simulink model "BVH2_App_Layer"  (Simulink 5.1)
settings: Solver=ode45  StartTime=0.0  StopTime=10.0  RelTol=1e-3
PreLoadFcn:
  | if exist('tl_preloadfcn','file'), tl_preloadfcn(gcs,95); end
PostLoadFcn:
  | if exist('tl_postloadfcn','file'), tl_postloadfcn(gcs,95); end
InitFcn:
  | if exist('tlds_start','file'), tlds_start(gcs); end
undefined symbols (not defined in the file): built, constant, Constant, DiscreteIntegrator, Gain, in, Logic, Product, Saturate, Sum, Switch
libraries: tllib x71, simulink x1
(part 3 of 4)

== system BVH2_App_Layer/BVH2_Appl_Layer/Subsystem/SFLogMain ==
  Stateflow Logger : tllib/Extras/Stateflow Logger  data=struct('date',730486)  sflogparam=struct('charts',[16 130 159 276 181 225 101 78 49],'sfblocks',{{'BVH2_App_Layer/BVH2_Appl_Layer/Subsystem/BVH2_Appl_Layer/Current_Analysis_High','BVH2_App_Layer/BVH2_Appl_Layer/Subsystem/BVH2_Appl_Layer/Current_Analysis_low','BVH2_App_Layer/BVH2_Appl_Layer/Subsystem/BVH2_Appl_Layer/Dry_Running','BVH2_App_Layer/BVH2_Appl_Layer/Subsystem/BVH2_Appl_Layer/Dry_RunningAlarm','BVH2_App_Layer/BVH2_Appl_Layer/Subsystem/BVH2_Appl_Layer/Motor_Stalled','BVH2_App_Layer/BVH2_Appl_Layer/Subsystem/BVH2_Appl_Layer/PWM_Detection','BVH2_App_Layer/BVH2_Appl_Layer/Subsystem/BVH2_Appl_Layer/Pic_etat_monitor','BVH2_App_Layer/BVH2_Appl_Layer/Subsystem/BVH2_Appl_Layer/Temperature_Alarm','BVH2_App_Layer/BVH2_Appl_Layer/Subsystem/BVH2_Appl_Layer/UbatHandling'}},'machines',15,'globallogopt',1,'modelname','BVH2_App_Layer','debugmodeactive',1)  flp_block=tldummylib/Stateflow Logger

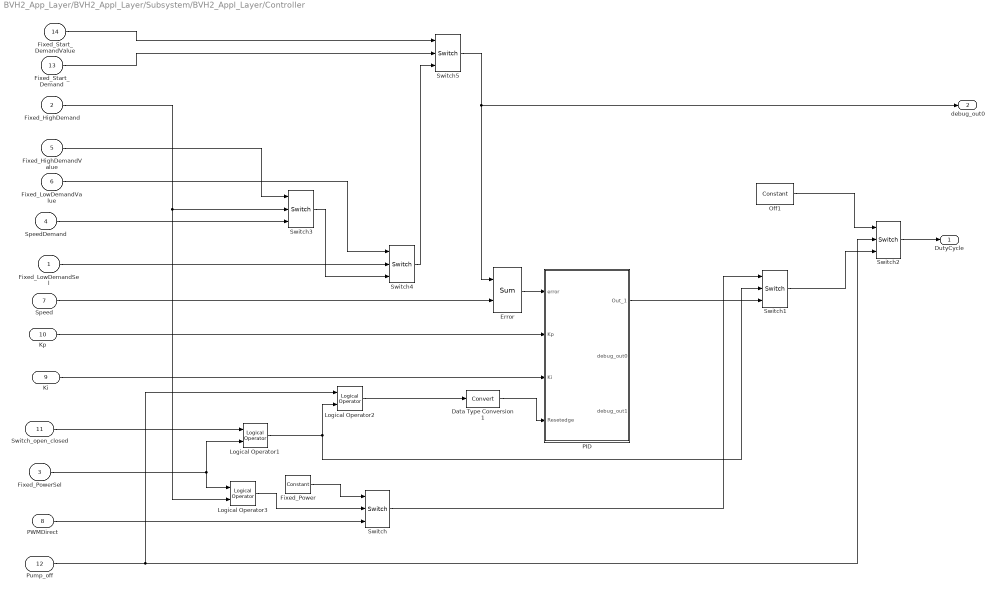
== system BVH2_App_Layer/BVH2_Appl_Layer/Subsystem/BVH2_Appl_Layer/Controller ==
  Fixed_LowDemandSel : Inport  PortDimensions=1  SampleTime=0.01
      settings: CopyFcn=tl_check_ports(gcbh);  NameChangeFcn=tl_check_ports(gcbh);
  Fixed_HighDemand : Inport  Port=2  PortDimensions=1  SampleTime=0.01
      settings: CopyFcn=tl_check_ports(gcbh);  NameChangeFcn=tl_check_ports(gcbh);
  Fixed_PowerSel : Inport  Port=3  PortDimensions=1  SampleTime=0.01
      settings: CopyFcn=tl_check_ports(gcbh);  NameChangeFcn=tl_check_ports(gcbh);
  SpeedDemand : Inport  Port=4  PortDimensions=1  SampleTime=0.01
      settings: CopyFcn=tl_check_ports(gcbh);  NameChangeFcn=tl_check_ports(gcbh);
  Fixed_HighDemandValue : Inport  Port=5  PortDimensions=1  SampleTime=0.01
      settings: CopyFcn=tl_check_ports(gcbh);  NameChangeFcn=tl_check_ports(gcbh);
  Fixed_LowDemandValue : Inport  Port=6  PortDimensions=1  SampleTime=0.01
      settings: CopyFcn=tl_check_ports(gcbh);  NameChangeFcn=tl_check_ports(gcbh);
  Speed : Inport  Port=7  PortDimensions=1  SampleTime=0.01
      settings: CopyFcn=tl_check_ports(gcbh);  NameChangeFcn=tl_check_ports(gcbh);
  PWMDirect : Inport  Port=8  PortDimensions=1  SampleTime=0.01
      settings: CopyFcn=tl_check_ports(gcbh);  NameChangeFcn=tl_check_ports(gcbh);
  Ki : Inport  Port=9  PortDimensions=1  SampleTime=0.01
      settings: CopyFcn=tl_check_ports(gcbh);  NameChangeFcn=tl_check_ports(gcbh);
  Kp : Inport  Port=10  PortDimensions=1  SampleTime=0.01
      settings: CopyFcn=tl_check_ports(gcbh);  NameChangeFcn=tl_check_ports(gcbh);
  Switch_open_closed : Inport  Port=11  PortDimensions=1  SampleTime=0.01
      settings: CopyFcn=tl_check_ports(gcbh);  NameChangeFcn=tl_check_ports(gcbh);
  Pump_off : Inport  Port=12  PortDimensions=1  SampleTime=0.01
      settings: CopyFcn=tl_check_ports(gcbh);  NameChangeFcn=tl_check_ports(gcbh);
  Fixed_Start_Demand : Inport  Port=13  PortDimensions=1  SampleTime=0.01
      settings: CopyFcn=tl_check_ports(gcbh);  NameChangeFcn=tl_check_ports(gcbh);
  Fixed_Start_DemandValue : Inport  Port=14  PortDimensions=1  SampleTime=0.01
      settings: CopyFcn=tl_check_ports(gcbh);  NameChangeFcn=tl_check_ports(gcbh);
  Data Type Conversion1 : DataTypeConversion  SaturateOnIntegerOverflow=on
  Error : tllib/Sum  data=struct('comment',struct('text','','placement',1),'logdata',struct('maxnumvals',inf,'plotchannels',1,'loggingmode',1,'channels',1),'output',struct('width',1,'name','$S_$B','unit','','type','Int16','offset',0,'max',NaN,'min',NaN,'freeze',1,'lsb',1,'arb',0,'class','default','address','','description','','autoscalingmode',1,'lowerheadroom',1,'upperheadroom',1,'headroomunit','bit','checkmin',0,'checkmax',0,'show',0,'variable','','scaling','','keepdatatype',1,'castoutput',0),'inputs','-+','date',735187.627440498,'scalingvalid',0)  lower_limit=1  upper_limit=-1  flp_block=built-in/Sum  help=|
      | Sum block of dSPACE TargetLink.
      | 
      | Output signal is equal to the sum of the input signals.
      | The list of signs is specified according to conventions for Simulink Sum blocks.
  Fixed_Power : tllib/Constant  Value=constant  ShowAdditionalParam=off  OutDataType=sfix(16)  ConRadixGroup=Use specified scaling  OutScaling=2^0  data=struct('comment',struct('text','','placement',1),'output',struct('width',1,'name','$S_$B','unit','','type','UInt16','offset',0,'max',NaN,'min',NaN,'freeze',1,'lsb',1,'arb',0,'class','CONST','address','','description','','value','202','tolerance',1,'show',0,'variable','','scaling','','keepdatatype',1),'date',734643.408264907,'scalingvalid',0)  constant=202  flp_block=built-in/Constant  help=|
      | Constant block of dSPACE TargetLink.
      | 
      | Output signal keeps the given constant value.
  Logical Operator1 : tllib/Logical Operator  data=struct('inputs','2','comment',struct('text','','placement',1),'logdata',struct('maxnumvals',inf,'plotchannels',[],'loggingmode',3,'channels',1),'operator','OR','output',struct('variable','','description','','name','$S_$B','address','','class','default','type','Bool','unit',''),'scalingvalid',0,'date',732283.44913765)  flp_block=built-in/Logic
  Logical Operator2 : tllib/Logical Operator  data=struct('inputs','2','comment',struct('text','','placement',1),'logdata',struct('maxnumvals',inf,'plotchannels',[],'loggingmode',3,'channels',1),'operator','OR','output',struct('variable','','description','','name','$S_$B','address','','class','default','type','Bool','unit',''),'scalingvalid',0,'date',732283.44913765)  flp_block=built-in/Logic
  Logical Operator3 : tllib/Logical Operator  data=struct('inputs','2','comment',struct('text','','placement',1),'logdata',struct('maxnumvals',inf,'plotchannels',[],'loggingmode',3,'channels',1),'operator','OR','output',struct('variable','','description','','name','$S_$B','address','','class','default','type','Bool','unit',''),'scalingvalid',0,'date',732283.44913765)  flp_block=built-in/Logic
  Off1 : tllib/Constant  Value=constant  ShowAdditionalParam=off  OutDataType=sfix(16)  ConRadixGroup=Use specified scaling  OutScaling=2^0  data=struct('comment',struct('text','','placement',1),'output',struct('width',1,'name','$S_$B','unit','','type','Int16','offset',0,'max',NaN,'min',NaN,'freeze',1,'lsb',1,'arb',0,'class','default','address','','description','','value','0','tolerance',1,'show',0,'variable','','scaling','','keepdatatype',1),'date',732121.729407349,'scalingvalid',0)  constant=0  flp_block=built-in/Constant  help=|
      | Constant block of dSPACE TargetLink.
      | 
      | Output signal keeps the given constant value.
  PID : Subsystem
  Switch{,3..5} (4 alike) : tllib/Switch  data=struct('comment',struct('text','','placement',1),'logdata',struct('maxnumvals',inf,'plotchannels',[],'loggingmode',3,'channels',1),'output',struct('variable','','description','','name','$S_$B','width',1,'address','','max',NaN,'min',NaN,'class','default','type','UInt16','scaling','','lsb',1,'offset',0,'arb',0,'freeze',1,'unit','','autoscalingmode',1,'lowerheadroom',1,'upperheadroom',1,'headroomunit','bit','keepdatatype',1,'checkmin',0,'checkmax',0,'castoutput',0,'show',0),'threshold',struct('variable','','description','','name','$S_$B_threshold','width',1,'address','','max',NaN,'min',NaN,'class','default','type','Int16','scaling','','lsb',1,'offset',0,'arb',0,'freeze',1,'unit','','keepdatatype',1,'value','0','scalar',0,'criteria',2),'scalingvalid',0,'date',732283.606852975)  threshold=0  flp_block=built-in/Switch
  Switch1 : tllib/Switch  data=struct('comment',struct('text','','placement',1),'logdata',struct('maxnumvals',inf,'plotchannels',[],'loggingmode',3,'channels',1),'output',struct('variable','','description','','name','$S_$B','width',1,'address','','max',NaN,'min',NaN,'class','default','type','UInt16','scaling','','lsb',1,'offset',0,'arb',0,'freeze',1,'unit','','autoscalingmode',1,'lowerheadroom',1,'upperheadroom',1,'headroomunit','bit','keepdatatype',1,'checkmin',0,'checkmax',0,'castoutput',0,'show',0),'threshold',struct('variable','','description','','name','$S_$B_threshold','width',1,'address','','max',NaN,'min',NaN,'class','default','type','Int16','scaling','','lsb',1,'offset',0,'arb',0,'freeze',1,'unit','','keepdatatype',1,'value','0','scalar',0,'criteria',2),'scalingvalid',0,'date',732283.593361933)  threshold=0  flp_block=built-in/Switch
  Switch2 : tllib/Switch  data=struct('comment',struct('text','','placement',1),'logdata',struct('maxnumvals',inf,'plotchannels',[],'loggingmode',3,'channels',1),'output',struct('variable','','description','','name','$S_$B','width',1,'address','','max',NaN,'min',NaN,'class','default','type','UInt16','scaling','','lsb',1,'offset',0,'arb',0,'freeze',1,'unit','','autoscalingmode',1,'lowerheadroom',1,'upperheadroom',1,'headroomunit','bit','keepdatatype',1,'checkmin',0,'checkmax',0,'castoutput',0,'show',0),'threshold',struct('variable','','description','','name','$S_$B_threshold','width',1,'address','','max',NaN,'min',NaN,'class','default','type','Int16','scaling','','lsb',1,'offset',0,'arb',0,'freeze',1,'unit','','keepdatatype',1,'value','0','scalar',0,'criteria',2),'scalingvalid',0,'date',732289.667383565)  threshold=0  flp_block=built-in/Switch
  DutyCycle : Outport
  debug_out0 : Outport  Port=2
  wires:
  Switch/1 -> Switch1/1
  Error/1 -> PID/1(error)
  Off1/1 -> Switch2/1
  PWMDirect/1 -> Switch/3
  Fixed_PowerSel/1 -> Logical Operator1/2, Logical Operator3/1
  Logical Operator1/1 -> Switch1/2, Logical Operator2/2
  Switch_open_closed/1 -> Logical Operator1/1
  Fixed_Power/1 -> Switch/1
  Pump_off/1 -> Switch2/2, Logical Operator2/1
  Switch1/1 -> Switch2/3
  Data Type Conversion1/1 -> PID/4(Resetedge)
  Logical Operator2/1 -> Data Type Conversion1/1
  Ki/1 -> PID/3(Ki)
  Kp/1 -> PID/2(Kp)
  PID/1(Out_1) -> Switch1/3
  Switch2/1 -> DutyCycle/1
  Speed/1 -> Error/2
  Fixed_HighDemand/1 -> Switch3/2, Logical Operator3/2
  Fixed_HighDemandValue/1 -> Switch3/1
  Logical Operator3/1 -> Switch/2
  Switch3/1 -> Switch4/3
  Fixed_LowDemandSel/1 -> Switch4/2
  Fixed_LowDemandValue/1 -> Switch4/1
  Fixed_Start_DemandValue/1 -> Switch5/1
  Fixed_Start_Demand/1 -> Switch5/2
  SpeedDemand/1 -> Switch3/3
  Switch4/1 -> Switch5/3
  Switch5/1 -> debug_out0/1, Error/1

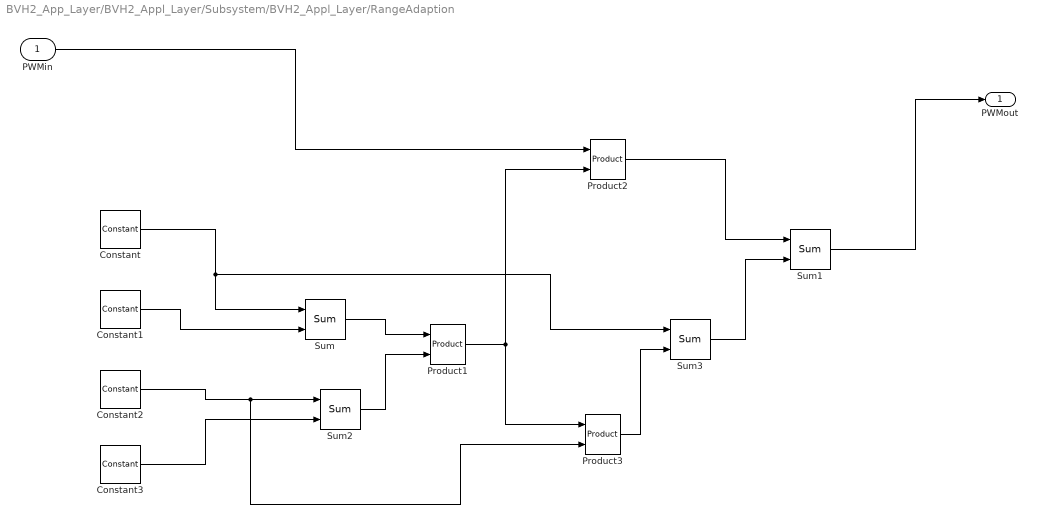
== system BVH2_App_Layer/BVH2_Appl_Layer/Subsystem/BVH2_Appl_Layer/RangeAdaption ==
  PWMin : Inport  PortDimensions=1  SampleTime=0.01
      settings: CopyFcn=tl_check_ports(gcbh);  NameChangeFcn=tl_check_ports(gcbh);
  Constant : tllib/Constant  Value=constant  ShowAdditionalParam=off  OutDataType=sfix(16)  ConRadixGroup=Use specified scaling  OutScaling=2^0  data=struct('comment',struct('text','','placement',1),'output',struct('variable','','description','','name','$S_$B','width',1,'address','','max',NaN,'min',NaN,'class','default','type','Int16','scaling','','lsb',1,'offset',0,'arb',0,'freeze',1,'unit','','keepdatatype',1,'value','200','tolerance',1,'show',0),'dt','inf','scalingvalid',0,'date',734591.489153391)  constant=200  flp_block=built-in/Constant
  Constant1 : tllib/Constant  Value=constant  ShowAdditionalParam=off  OutDataType=sfix(16)  ConRadixGroup=Use specified scaling  OutScaling=2^0  data=struct('comment',struct('text','','placement',1),'output',struct('variable','','description','','name','$S_$B','width',1,'address','','max',NaN,'min',NaN,'class','default','type','Int16','scaling','','lsb',1,'offset',0,'arb',0,'freeze',1,'unit','','keepdatatype',1,'value','60','tolerance',1,'show',0),'dt','inf','scalingvalid',0,'date',734591.489234537)  constant=60  flp_block=built-in/Constant
  Constant2 : tllib/Constant  Value=constant  ShowAdditionalParam=off  OutDataType=sfix(16)  ConRadixGroup=Use specified scaling  OutScaling=2^0  data=struct('comment',struct('text','','placement',1),'output',struct('variable','','description','','name','$S_$B','width',1,'address','','max',NaN,'min',NaN,'class','default','type','Int16','scaling','','lsb',1,'offset',0,'arb',0,'freeze',1,'unit','','keepdatatype',1,'value','190','tolerance',1,'show',0),'dt','inf','scalingvalid',0,'date',734591.488197627)  constant=190  flp_block=built-in/Constant
  Constant3 : tllib/Constant  Value=constant  ShowAdditionalParam=off  OutDataType=sfix(16)  ConRadixGroup=Use specified scaling  OutScaling=2^0  data=struct('comment',struct('text','','placement',1),'output',struct('variable','','description','','name','$S_$B','width',1,'address','','max',NaN,'min',NaN,'class','default','type','Int16','scaling','','lsb',1,'offset',0,'arb',0,'freeze',1,'unit','','keepdatatype',1,'value','30','tolerance',1,'show',0),'dt','inf','scalingvalid',0,'date',734591.48794713)  constant=30  flp_block=built-in/Constant
  Product1 : tllib/Product  data=struct('comment',struct('text','','placement',1),'logdata',struct('maxnumvals',inf,'plotchannels',[],'loggingmode',3,'channels',1),'output',struct('width',1,'name','$S_$B','unit','','type','UInt16','offset',0,'max',NaN,'min',NaN,'freeze',1,'lsb',2^-8,'arb',0,'class','default','address','','description','','autoscalingmode',1,'lowerheadroom',0,'upperheadroom',1,'headroomunit','bit','checkmin',0,'checkmax',0,'show',0,'variable','','scaling','','keepdatatype',1,'castoutput',0),'inputs','*/','exceptionhandling',1,'date',734591.551719815,'scalingvalid',0)  lower_limit=1  upper_limit=-1  flp_block=built-in/Product  help=|
      | Product block of dSPACE TargetLink.
      | 
      | Output signal is equal to the product of the input signals. The input ports are specified according to conventions for Simulink Product blocks.
  Product2 : tllib/Product  data=struct('comment',struct('text','','placement',1),'logdata',struct('maxnumvals',inf,'plotchannels',[],'loggingmode',3,'channels',1),'output',struct('width',1,'name','$S_$B','unit','','type','UInt16','offset',0,'max',NaN,'min',NaN,'freeze',1,'lsb',1,'arb',0,'class','default','address','','description','','autoscalingmode',1,'lowerheadroom',0,'upperheadroom',1,'headroomunit','bit','checkmin',0,'checkmax',0,'show',0,'variable','','scaling','','keepdatatype',1,'castoutput',0),'inputs','**','exceptionhandling',1,'date',732813.755751852,'scalingvalid',0)  lower_limit=1  upper_limit=-1  flp_block=built-in/Product  help=|
      | Product block of dSPACE TargetLink.
      | 
      | Output signal is equal to the product of the input signals. The input ports are specified according to conventions for Simulink Product blocks.
  Product3 : tllib/Product  data=struct('comment',struct('text','','placement',1),'logdata',struct('maxnumvals',inf,'plotchannels',[],'loggingmode',3,'channels',1),'output',struct('width',1,'name','$S_$B','unit','','type','UInt16','offset',0,'max',NaN,'min',NaN,'freeze',1,'lsb',1,'arb',0,'class','default','address','','description','','autoscalingmode',1,'lowerheadroom',0,'upperheadroom',1,'headroomunit','bit','checkmin',0,'checkmax',0,'show',0,'variable','','scaling','','keepdatatype',1,'castoutput',0),'inputs','**','exceptionhandling',1,'date',732813.755751852,'scalingvalid',0)  lower_limit=1  upper_limit=-1  flp_block=built-in/Product  help=|
      | Product block of dSPACE TargetLink.
      | 
      | Output signal is equal to the product of the input signals. The input ports are specified according to conventions for Simulink Product blocks.
  Sum : tllib/Sum  data=struct('comment',struct('text','','placement',1),'logdata',struct('maxnumvals',inf,'plotchannels',[],'loggingmode',3,'channels',1),'output',struct('variable','','description','','name','$S_$B','width',1,'address','','max',NaN,'min',NaN,'class','default','type','Int16','scaling','','lsb',1,'offset',0,'arb',0,'freeze',1,'unit','','autoscalingmode',1,'lowerheadroom',1,'upperheadroom',1,'headroomunit','bit','keepdatatype',1,'checkmin',0,'checkmax',0,'castoutput',0,'show',0),'inputs','+-','scalingvalid',0,'date',733019.586384155)  flp_block=built-in/Sum
  Sum1 : tllib/Sum  data=struct('comment',struct('text','','placement',1),'logdata',struct('maxnumvals',inf,'plotchannels',[],'loggingmode',3,'channels',1),'output',struct('variable','','description','','name','$S_$B','width',1,'address','','max',NaN,'min',NaN,'class','default','type','Int16','scaling','','lsb',1,'offset',0,'arb',0,'freeze',1,'unit','','autoscalingmode',1,'lowerheadroom',1,'upperheadroom',1,'headroomunit','bit','keepdatatype',1,'checkmin',0,'checkmax',0,'castoutput',0,'show',0),'inputs','++','scalingvalid',0,'date',734591.551219225)  flp_block=built-in/Sum
  Sum2 : tllib/Sum  data=struct('comment',struct('text','','placement',1),'logdata',struct('maxnumvals',inf,'plotchannels',[],'loggingmode',3,'channels',1),'output',struct('variable','','description','','name','$S_$B','width',1,'address','','max',NaN,'min',NaN,'class','default','type','Int16','scaling','','lsb',1,'offset',0,'arb',0,'freeze',1,'unit','','autoscalingmode',1,'lowerheadroom',1,'upperheadroom',1,'headroomunit','bit','keepdatatype',1,'checkmin',0,'checkmax',0,'castoutput',0,'show',0),'inputs','+-','scalingvalid',0,'date',733019.586384155)  flp_block=built-in/Sum
  Sum3 : tllib/Sum  data=struct('comment',struct('text','','placement',1),'logdata',struct('maxnumvals',inf,'plotchannels',[],'loggingmode',3,'channels',1),'output',struct('variable','','description','','name','$S_$B','width',1,'address','','max',NaN,'min',NaN,'class','default','type','Int16','scaling','','lsb',1,'offset',0,'arb',0,'freeze',1,'unit','','autoscalingmode',1,'lowerheadroom',1,'upperheadroom',1,'headroomunit','bit','keepdatatype',1,'checkmin',0,'checkmax',0,'castoutput',0,'show',0),'inputs','+-','scalingvalid',0,'date',733019.586384155)  flp_block=built-in/Sum
  PWMout : Outport
  wires:
  PWMin/1 -> Product2/1
  Product2/1 -> Sum1/1
  Constant/1 -> Sum/1, Sum3/1
  Constant1/1 -> Sum/2
  Sum/1 -> Product1/1
  Constant2/1 -> Sum2/1, Product3/2
  Constant3/1 -> Sum2/2
  Sum2/1 -> Product1/2
  Product1/1 -> Product2/2, Product3/1
  Product3/1 -> Sum3/2
  Sum3/1 -> Sum1/2
  Sum1/1 -> PWMout/1

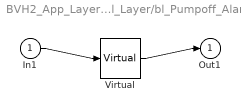
== system BVH2_App_Layer/BVH2_Appl_Layer/Subsystem/BVH2_Appl_Layer/bl_Pumpoff_Alarm ==
  In1 : Inport
  Virtual : tllib/Virtual  SimViewingDevice=off  DataTypeOverride=UseLocalSettings  MinMaxOverflowLogging=UseLocalSettings
      settings: Permissions=ReadWrite  RTWFcnNameOpts=Auto  RTWFileNameOpts=Auto
  Out1 : Outport
  wires:
  In1/1 -> Virtual/1
  Virtual/1 -> Out1/1

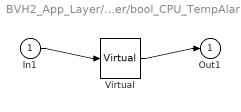
== system BVH2_App_Layer/BVH2_Appl_Layer/Subsystem/BVH2_Appl_Layer/bool_CPU_TempAlarm ==
  In1 : Inport
  Virtual : tllib/Virtual  SimViewingDevice=off  DataTypeOverride=UseLocalSettings  MinMaxOverflowLogging=UseLocalSettings
      settings: Permissions=ReadWrite  RTWFcnNameOpts=Auto  RTWFileNameOpts=Auto
  Out1 : Outport
  wires:
  In1/1 -> Virtual/1
  Virtual/1 -> Out1/1

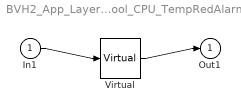
== system BVH2_App_Layer/BVH2_Appl_Layer/Subsystem/BVH2_Appl_Layer/bool_CPU_TempRedAlarm ==
  In1 : Inport
  Virtual : tllib/Virtual  SimViewingDevice=off  DataTypeOverride=UseLocalSettings  MinMaxOverflowLogging=UseLocalSettings
      settings: Permissions=ReadWrite  RTWFcnNameOpts=Auto  RTWFileNameOpts=Auto
  Out1 : Outport
  wires:
  In1/1 -> Virtual/1
  Virtual/1 -> Out1/1

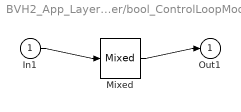
== system BVH2_App_Layer/BVH2_Appl_Layer/Subsystem/BVH2_Appl_Layer/bool_ControlLoopMode ==
  In1 : Inport
  Mixed : tllib/Mixed  SimViewingDevice=off  DataTypeOverride=UseLocalSettings  MinMaxOverflowLogging=UseLocalSettings
      settings: Permissions=ReadWrite  RTWFcnNameOpts=Auto  RTWFileNameOpts=Auto
  Out1 : Outport
  wires:
  In1/1 -> Mixed/1
  Mixed/1 -> Out1/1

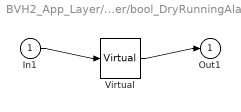
== system BVH2_App_Layer/BVH2_Appl_Layer/Subsystem/BVH2_Appl_Layer/bool_DryRunningAlarm ==
  In1 : Inport
  Virtual : tllib/Virtual  SimViewingDevice=off  DataTypeOverride=UseLocalSettings  MinMaxOverflowLogging=UseLocalSettings
      settings: Permissions=ReadWrite  RTWFcnNameOpts=Auto  RTWFileNameOpts=Auto
  Out1 : Outport
  wires:
  In1/1 -> Virtual/1
  Virtual/1 -> Out1/1

== system BVH2_App_Layer/BVH2_Appl_Layer/Subsystem/BVH2_Appl_Layer/bool_HighCurrentAlarm ==
  In1 : Inport
  Virtual : tllib/Virtual  SimViewingDevice=off  DataTypeOverride=UseLocalSettings  MinMaxOverflowLogging=UseLocalSettings
      settings: Permissions=ReadWrite  RTWFcnNameOpts=Auto  RTWFileNameOpts=Auto
  Out1 : Outport
  wires:
  In1/1 -> Virtual/1
  Virtual/1 -> Out1/1

== system BVH2_App_Layer/BVH2_Appl_Layer/Subsystem/BVH2_Appl_Layer/bool_MotorStalled ==
  In1 : Inport
  Virtual : tllib/Virtual  SimViewingDevice=off  DataTypeOverride=UseLocalSettings  MinMaxOverflowLogging=UseLocalSettings
      settings: Permissions=ReadWrite  RTWFcnNameOpts=Auto  RTWFileNameOpts=Auto
  Out1 : Outport
  wires:
  In1/1 -> Virtual/1
  Virtual/1 -> Out1/1

== system BVH2_App_Layer/BVH2_Appl_Layer/Subsystem/BVH2_Appl_Layer/bool_PIC_Alarm ==
  In1 : Inport
  Virtual : tllib/Virtual  SimViewingDevice=off  DataTypeOverride=UseLocalSettings  MinMaxOverflowLogging=UseLocalSettings
      settings: Permissions=ReadWrite  RTWFcnNameOpts=Auto  RTWFileNameOpts=Auto
  Out1 : Outport
  wires:
  In1/1 -> Virtual/1
  Virtual/1 -> Out1/1

== system BVH2_App_Layer/BVH2_Appl_Layer/Subsystem/BVH2_Appl_Layer/bool_PWMin_Freq_err_Alarm ==
  In1 : Inport
  Virtual : tllib/Virtual  SimViewingDevice=off  DataTypeOverride=UseLocalSettings  MinMaxOverflowLogging=UseLocalSettings
      settings: Permissions=ReadWrite  RTWFcnNameOpts=Auto  RTWFileNameOpts=Auto
  Out1 : Outport
  wires:
  In1/1 -> Virtual/1
  Virtual/1 -> Out1/1

== system BVH2_App_Layer/BVH2_Appl_Layer/Subsystem/BVH2_Appl_Layer/bool_PWMin_err_Alarm ==
  In1 : Inport
  Virtual : tllib/Virtual  SimViewingDevice=off  DataTypeOverride=UseLocalSettings  MinMaxOverflowLogging=UseLocalSettings
      settings: Permissions=ReadWrite  RTWFcnNameOpts=Auto  RTWFileNameOpts=Auto
  Out1 : Outport
  wires:
  In1/1 -> Virtual/1
  Virtual/1 -> Out1/1

== system BVH2_App_Layer/BVH2_Appl_Layer/Subsystem/BVH2_Appl_Layer/bool_StalledMotorStop ==
  In1 : Inport
  Virtual : tllib/Virtual  SimViewingDevice=off  DataTypeOverride=UseLocalSettings  MinMaxOverflowLogging=UseLocalSettings
      settings: Permissions=ReadWrite  RTWFcnNameOpts=Auto  RTWFileNameOpts=Auto
  Out1 : Outport
  wires:
  In1/1 -> Virtual/1
  Virtual/1 -> Out1/1

== system BVH2_App_Layer/BVH2_Appl_Layer/Subsystem/BVH2_Appl_Layer/bool_UbatAlarm ==
  In1 : Inport
  Virtual : tllib/Virtual  SimViewingDevice=off  DataTypeOverride=UseLocalSettings  MinMaxOverflowLogging=UseLocalSettings
      settings: Permissions=ReadWrite  RTWFcnNameOpts=Auto  RTWFileNameOpts=Auto
  Out1 : Outport
  wires:
  In1/1 -> Virtual/1
  Virtual/1 -> Out1/1

== system BVH2_App_Layer/BVH2_Appl_Layer/Subsystem/BVH2_Appl_Layer/bool_mat_currAlarm_bldc ==
  In1 : Inport
  Mixed : tllib/Mixed  SimViewingDevice=off  DataTypeOverride=UseLocalSettings  MinMaxOverflowLogging=UseLocalSettings
      settings: Permissions=ReadWrite  RTWFcnNameOpts=Auto  RTWFileNameOpts=Auto
  Out1 : Outport
  wires:
  In1/1 -> Mixed/1
  Mixed/1 -> Out1/1

== system BVH2_App_Layer/BVH2_Appl_Layer/Subsystem/BVH2_Appl_Layer/bool_mat_pic_etat ==
  In1 : Inport
  Mixed : tllib/Mixed  SimViewingDevice=off  DataTypeOverride=UseLocalSettings  MinMaxOverflowLogging=UseLocalSettings
      settings: Permissions=ReadWrite  RTWFcnNameOpts=Auto  RTWFileNameOpts=Auto
  Out1 : Outport
  wires:
  In1/1 -> Mixed/1
  Mixed/1 -> Out1/1

== system BVH2_App_Layer/BVH2_Appl_Layer/Subsystem/BVH2_Appl_Layer/bool_start_demand_mat ==
  In1 : Inport
  Mixed : tllib/Mixed  SimViewingDevice=off  DataTypeOverride=UseLocalSettings  MinMaxOverflowLogging=UseLocalSettings
      settings: Permissions=ReadWrite  RTWFcnNameOpts=Auto  RTWFileNameOpts=Auto
  Out1 : Outport
  wires:
  In1/1 -> Mixed/1
  Mixed/1 -> Out1/1

== system BVH2_App_Layer/BVH2_Appl_Layer/Subsystem/BVH2_Appl_Layer/ui16_Current_Thresh ==
  In1 : Inport
  Mixed : tllib/Mixed  SimViewingDevice=off  DataTypeOverride=UseLocalSettings  MinMaxOverflowLogging=UseLocalSettings
      settings: Permissions=ReadWrite  RTWFcnNameOpts=Auto  RTWFileNameOpts=Auto
  Out1 : Outport
  wires:
  In1/1 -> Mixed/1
  Mixed/1 -> Out1/1

== system BVH2_App_Layer/BVH2_Appl_Layer/Subsystem/BVH2_Appl_Layer/ui16_PWM_Freq_mat ==
  In1 : Inport
  Mixed : tllib/Mixed  SimViewingDevice=off  DataTypeOverride=UseLocalSettings  MinMaxOverflowLogging=UseLocalSettings
      settings: Permissions=ReadWrite  RTWFcnNameOpts=Auto  RTWFileNameOpts=Auto
  Out1 : Outport
  wires:
  In1/1 -> Mixed/1
  Mixed/1 -> Out1/1

== system BVH2_App_Layer/BVH2_Appl_Layer/Subsystem/BVH2_Appl_Layer/ui16_Speed_demand_mat ==
  In1 : Inport
  Mixed : tllib/Mixed  SimViewingDevice=off  DataTypeOverride=UseLocalSettings  MinMaxOverflowLogging=UseLocalSettings
      settings: Permissions=ReadWrite  RTWFcnNameOpts=Auto  RTWFileNameOpts=Auto
  Out1 : Outport
  wires:
  In1/1 -> Mixed/1
  Mixed/1 -> Out1/1

== system BVH2_App_Layer/BVH2_Appl_Layer/Subsystem/BVH2_Appl_Layer/ui16_Speed_demand_mat_Max ==
  In1 : Inport
  Mixed : tllib/Mixed  SimViewingDevice=off  DataTypeOverride=UseLocalSettings  MinMaxOverflowLogging=UseLocalSettings
      settings: Permissions=ReadWrite  RTWFcnNameOpts=Auto  RTWFileNameOpts=Auto
  Out1 : Outport
  wires:
  In1/1 -> Mixed/1
  Mixed/1 -> Out1/1

== system BVH2_App_Layer/BVH2_Appl_Layer/Subsystem/BVH2_Appl_Layer/ui16_Speed_demand_mat_min ==
  In1 : Inport
  Mixed : tllib/Mixed  SimViewingDevice=off  DataTypeOverride=UseLocalSettings  MinMaxOverflowLogging=UseLocalSettings
      settings: Permissions=ReadWrite  RTWFcnNameOpts=Auto  RTWFileNameOpts=Auto
  Out1 : Outport
  wires:
  In1/1 -> Mixed/1
  Mixed/1 -> Out1/1

== system BVH2_App_Layer/BVH2_Appl_Layer/Subsystem/BVH2_Appl_Layer/ui16_Speed_mat ==
  In1 : Inport
  Mixed : tllib/Mixed  SimViewingDevice=off  DataTypeOverride=UseLocalSettings  MinMaxOverflowLogging=UseLocalSettings
      settings: Permissions=ReadWrite  RTWFcnNameOpts=Auto  RTWFileNameOpts=Auto
  Out1 : Outport
  wires:
  In1/1 -> Mixed/1
  Mixed/1 -> Out1/1

== system BVH2_App_Layer/BVH2_Appl_Layer/Subsystem/BVH2_Appl_Layer/ui16_dryRun_Thresh ==
  In1 : Inport
  Mixed : tllib/Mixed  SimViewingDevice=off  DataTypeOverride=UseLocalSettings  MinMaxOverflowLogging=UseLocalSettings
      settings: Permissions=ReadWrite  RTWFcnNameOpts=Auto  RTWFileNameOpts=Auto
  Out1 : Outport
  wires:
  In1/1 -> Mixed/1
  Mixed/1 -> Out1/1

== system BVH2_App_Layer/BVH2_Appl_Layer/Subsystem/BVH2_Appl_Layer/ui16_mat_Current ==
  In1 : Inport
  Mixed : tllib/Mixed  SimViewingDevice=off  DataTypeOverride=UseLocalSettings  MinMaxOverflowLogging=UseLocalSettings
      settings: Permissions=ReadWrite  RTWFcnNameOpts=Auto  RTWFileNameOpts=Auto
  Out1 : Outport
  wires:
  In1/1 -> Mixed/1
  Mixed/1 -> Out1/1

== system BVH2_App_Layer/BVH2_Appl_Layer/Subsystem/BVH2_Appl_Layer/ui16_mat_inpTemp ==
  In1 : Inport
  Mixed : tllib/Mixed  SimViewingDevice=off  DataTypeOverride=UseLocalSettings  MinMaxOverflowLogging=UseLocalSettings
      settings: Permissions=ReadWrite  RTWFcnNameOpts=Auto  RTWFileNameOpts=Auto
  Out1 : Outport
  wires:
  In1/1 -> Mixed/1
  Mixed/1 -> Out1/1

== system BVH2_App_Layer/BVH2_Appl_Layer/Subsystem/BVH2_Appl_Layer/ui8_BattVolt_mat ==
  In1 : Inport
  Mixed : tllib/Mixed  SimViewingDevice=off  DataTypeOverride=UseLocalSettings  MinMaxOverflowLogging=UseLocalSettings
      settings: Permissions=ReadWrite  RTWFcnNameOpts=Auto  RTWFileNameOpts=Auto
  Out1 : Outport
  wires:
  In1/1 -> Mixed/1
  Mixed/1 -> Out1/1

== system BVH2_App_Layer/BVH2_Appl_Layer/Subsystem/BVH2_Appl_Layer/ui8_Ki_mat ==
  In1 : Inport
  Mixed : tllib/Mixed  SimViewingDevice=off  DataTypeOverride=UseLocalSettings  MinMaxOverflowLogging=UseLocalSettings
      settings: Permissions=ReadWrite  RTWFcnNameOpts=Auto  RTWFileNameOpts=Auto
  Out1 : Outport
  wires:
  In1/1 -> Mixed/1
  Mixed/1 -> Out1/1

== system BVH2_App_Layer/BVH2_Appl_Layer/Subsystem/BVH2_Appl_Layer/ui8_Kp_mat ==
  In1 : Inport
  Mixed : tllib/Mixed  SimViewingDevice=off  DataTypeOverride=UseLocalSettings  MinMaxOverflowLogging=UseLocalSettings
      settings: Permissions=ReadWrite  RTWFcnNameOpts=Auto  RTWFileNameOpts=Auto
  Out1 : Outport
  wires:
  In1/1 -> Mixed/1
  Mixed/1 -> Out1/1

== system BVH2_App_Layer/BVH2_Appl_Layer/Subsystem/BVH2_Appl_Layer/ui8_PWM_dc_mat ==
  In1 : Inport
  Mixed : tllib/Mixed  SimViewingDevice=off  DataTypeOverride=UseLocalSettings  MinMaxOverflowLogging=UseLocalSettings
      settings: Permissions=ReadWrite  RTWFcnNameOpts=Auto  RTWFileNameOpts=Auto
  Out1 : Outport
  wires:
  In1/1 -> Mixed/1
  Mixed/1 -> Out1/1

== system BVH2_App_Layer/BVH2_Appl_Layer/Subsystem/BVH2_Appl_Layer/ui8_ResetMatlab ==
  In1 : Inport
  Mixed : tllib/Mixed  SimViewingDevice=off  DataTypeOverride=UseLocalSettings  MinMaxOverflowLogging=UseLocalSettings
      settings: Permissions=ReadWrite  RTWFcnNameOpts=Auto  RTWFileNameOpts=Auto
  Out1 : Outport
  wires:
  In1/1 -> Mixed/1
  Mixed/1 -> Out1/1

== system BVH2_App_Layer/BVH2_Appl_Layer/Subsystem/BVH2_Appl_Layer/ui8_debug_out0 ==
  In1 : Inport
  Virtual : tllib/Virtual  SimViewingDevice=off  DataTypeOverride=UseLocalSettings  MinMaxOverflowLogging=UseLocalSettings
      settings: Permissions=ReadWrite  RTWFcnNameOpts=Auto  RTWFileNameOpts=Auto
  Out1 : Outport
  wires:
  In1/1 -> Virtual/1
  Virtual/1 -> Out1/1

== system BVH2_App_Layer/BVH2_Appl_Layer/Subsystem/BVH2_Appl_Layer/ui8_duty_cycle_mat ==
  In1 : Inport
  Virtual : tllib/Virtual  SimViewingDevice=off  DataTypeOverride=UseLocalSettings  MinMaxOverflowLogging=UseLocalSettings
      settings: Permissions=ReadWrite  RTWFcnNameOpts=Auto  RTWFileNameOpts=Auto
  Out1 : Outport
  wires:
  In1/1 -> Virtual/1
  Virtual/1 -> Out1/1

== system BVH2_App_Layer/BVH2_Appl_Layer/Subsystem/BVH2_Appl_Layer/ui8_fixed_start_speed_mat ==
  In1 : Inport
  Mixed : tllib/Mixed  SimViewingDevice=off  DataTypeOverride=UseLocalSettings  MinMaxOverflowLogging=UseLocalSettings
      settings: Permissions=ReadWrite  RTWFcnNameOpts=Auto  RTWFileNameOpts=Auto
  Out1 : Outport
  wires:
  In1/1 -> Mixed/1
  Mixed/1 -> Out1/1

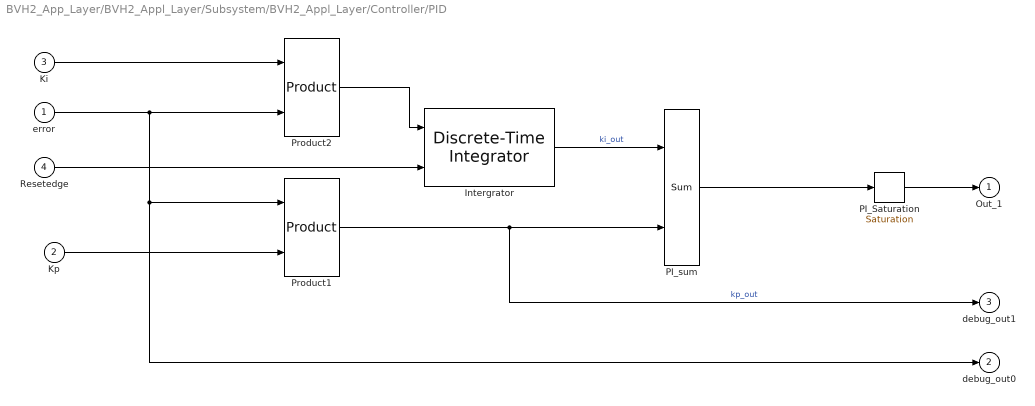
== system BVH2_App_Layer/BVH2_Appl_Layer/Subsystem/BVH2_Appl_Layer/Controller/PID ==
  error : Inport
  Kp : Inport  Port=2
  Ki : Inport  Port=3
  Resetedge : Inport  Port=4
  Intergrator : tllib/Discrete-Time Integrator  data=struct('comment',struct('text','','placement',1),'logdata',struct('maxnumvals',inf,'plotchannels',[],'loggingmode',3,'channels',1),'output',struct('width',1,'name','$S_$B','unit','','type','Int16','offset',0,'max',NaN,'min',NaN,'freeze',1,'lsb',1,'arb',0,'class','default','address','','description','','autoscalingmode',1,'lowerheadroom',1,'upperheadroom',1,'headroomunit','bit','show',0,'variable','','scaling','','keepdatatype',1,'castoutput',1),'state',struct('width',1,'name','X_$S_$B','unit','','type','Int16','offset',0,'max',NaN,'min',NaN,'freeze',1,'lsb',1,'arb',0,'class','default','address','','description','','externalreset',4,'initialconditionsource',1,'showsaturation',0,'initial','100','variable','','scaling',''),'input',struct('name','U_$S_$B','unit','','class','default','address','','description','','variable',''),'lowerlimit',struct('width',1,'name','$S_$B_lower','unit','','type','Int16','offset',0,'max',NaN,'min',NaN,'freeze',1,'lsb',1,'arb',0,'class','default','address','','description','','value','40','variable','','scaling','','keepdatatype',1),'upperlimit',struct('width',1,'name','$S_$B_upper','unit','','type','Int16','offset',0,'max',NaN,'min',NaN,'freeze',1,'lsb',1,'arb',0,'class','default','address','','description','','value','202','variable','','scaling','','keepdatatype',1),'integrationmethod',1,'dt','0.01','date',734772.541916007,'scalingvalid',0)  dt=0.01  lower_limit=40  upper_limit=202  X0=100  flp_block=built-in/DiscreteIntegrator  help=|
      | Discrete Integrator block of dSPACE TargetLink.
      | Forward and backward rectangular and trapezoidal integration are supported.
      | 
      | Note that this block is not vectorized.
  PI_Saturation : tllib/Saturation  data=struct('comment',struct('text','','placement',1),'logdata',struct('maxnumvals',inf,'plotchannels',[],'loggingmode',3,'channels',1),'output',struct('width',1,'name','$S_$B','unit','','type','UInt16','offset',0,'max',NaN,'min',NaN,'freeze',1,'lsb',1,'arb',0,'class','default','address','','description','','autoscalingmode',1,'lowerheadroom',0,'upperheadroom',1,'headroomunit','bit','show',0,'variable','','scaling','','keepdatatype',1,'castoutput',0),'lowerlimit',struct('width',1,'name','$S_$B_lower','unit','','type','Int16','offset',0,'max',NaN,'min',NaN,'freeze',1,'lsb',1,'arb',0,'class','default','address','','description','','value','40','scalar',0,'variable','','scaling','','keepdatatype',1),'upperlimit',struct('width',1,'name','$S_$B_upper','unit','','type','Int16','offset',0,'max',NaN,'min',NaN,'freeze',1,'lsb',1,'arb',0,'class','default','address','','description','','value','202','scalar',0,'variable','','scaling','','keepdatatype',1),'date',734772.541953438,'scalingvalid',0)  lower_limit=40  upper_limit=202  flp_block=built-in/Saturate  help=|
      | Saturation block of dSPACE TargetLink.
      | 
      | The Saturation block saturates its input to the given upper and lower limit.
  PI_sum : tllib/Sum  data=struct('comment',struct('text','','placement',1),'logdata',struct('maxnumvals',inf,'plotchannels',[],'loggingmode',3,'channels',1),'output',struct('width',1,'name','$S_$B','unit','','type','Int16','offset',0,'max',NaN,'min',NaN,'freeze',1,'lsb',1,'arb',0,'class','default','address','','description','','autoscalingmode',1,'lowerheadroom',1,'upperheadroom',1,'headroomunit','bit','checkmin',0,'checkmax',0,'show',0,'variable','','scaling','','keepdatatype',1,'castoutput',0),'inputs','++','date',734643.573882407,'scalingvalid',0)  lower_limit=1  upper_limit=-1  flp_block=built-in/Sum  help=|
      | Sum block of dSPACE TargetLink.
      | 
      | Output signal is equal to the sum of the input signals.
      | The list of signs is specified according to conventions for Simulink Sum blocks.
  Product1 : tllib/Product  data=struct('comment',struct('text','','placement',1),'logdata',struct('maxnumvals',inf,'plotchannels',[],'loggingmode',3,'channels',1),'output',struct('width',1,'name','$S_$B','unit','','type','Int16','offset',0,'max',NaN,'min',NaN,'freeze',1,'lsb',1,'arb',0,'class','default','address','','description','','autoscalingmode',1,'lowerheadroom',1,'upperheadroom',1,'headroomunit','bit','checkmin',0,'checkmax',0,'show',0,'variable','','scaling','','keepdatatype',1,'castoutput',0),'inputs','**','exceptionhandling',1,'date',734643.573922176,'scalingvalid',0)  lower_limit=1  upper_limit=-1  flp_block=built-in/Product  help=|
      | Product block of dSPACE TargetLink.
      | 
      | Output signal is equal to the product of the input signals. The input ports are specified according to conventions for Simulink Product blocks.
  Product2 : tllib/Product  data=struct('comment',struct('text','','placement',1),'logdata',struct('maxnumvals',inf,'plotchannels',[],'loggingmode',3,'channels',1),'output',struct('width',1,'name','$S_$B','unit','','type','Int16','offset',0,'max',NaN,'min',NaN,'freeze',1,'lsb',2^-3,'arb',0,'class','default','address','','description','','autoscalingmode',1,'lowerheadroom',1,'upperheadroom',1,'headroomunit','bit','checkmin',0,'checkmax',0,'show',0,'variable','','scaling','','keepdatatype',1,'castoutput',0),'inputs','**','exceptionhandling',1,'date',734713.639518102,'scalingvalid',0)  lower_limit=1  upper_limit=-1  flp_block=built-in/Product  help=|
      | Product block of dSPACE TargetLink.
      | 
      | Output signal is equal to the product of the input signals. The input ports are specified according to conventions for Simulink Product blocks.
  Out_1 : Outport  InitialOutput=0
  debug_out0 : Outport  Port=2  InitialOutput=0
  debug_out1 : Outport  Port=3  InitialOutput=0
  wires:
  error/1 -> Product2/2, Product1/1, debug_out0/1
  Product2/1 -> Intergrator/1
  Intergrator/1 -> PI_sum/1  "ki_out"
  Kp/1 -> Product1/2
  Ki/1 -> Product2/1
  PI_Saturation/1 -> Out_1/1
  Resetedge/1 -> Intergrator/2
  PI_sum/1 -> PI_Saturation/1
  Product1/1 -> PI_sum/2, debug_out1/1  "kp_out"

== stateflow chart BVH2_Appl_Layer/Subsystem/BVH2_Appl_Layer/Current_Analysis_High ==
  state redState
    entry:
    StateCnt=0;
    oShutoff = 1;
    oCurrentAlarm = 1;
    during:
    StateCnt++;
  state CntOverCurrent
    entry:
    StateCnt = 0 ;
    during:
    StateCnt++ ;
  state greenState
    entry:
    oShutoff  = 0 ;
    oCurrentAlarm = 1;
    StateCnt = 0;
    during:
    StateCnt++;
  state Wait
    entry:
    StateCnt = 0;
    during:
    StateCnt++;
  state Alarm_Off
    entry:
    oShutoff  = 0 ;
    oCurrentAlarm = 0;
    RestartCounter = 0
  state Reset
    entry:
    StateCnt=0;
    RestartCounter = 0;
    during:
    StateCnt++ ;
  note: /* When Alarm for CurrentLimit is set by BLDC,
      | the pump is stopped and the current alarm is set while this alarm is not removed.
      | Until this alarm is removed, the pump can restart 1s later and
      | the current alarm is removed 500ms after*/
  state RestartCounter
    entry:
    RestartCounter ++;
  (junction 13) -> CntOverCurrent : [iAlarm==1]
  (default) -> Reset : [iReset==1]
  redState -> Wait : [iAlarm == 0]
  (junction 11) -> redState : [StateCnt  > 1]
  CntOverCurrent -> (junction 11)
  (junction 11) -> greenState : [iAlarm == 0]
  (junction 12) -> RestartCounter : [StateCnt  > 200 ]
  Wait -> (junction 12)
  (junction 12) -> redState : [iAlarm == 1]
  Alarm_Off -> (junction 13)
  greenState -> (junction 13)
  (junction 13) -> Alarm_Off : [ StateCnt  > 100 ]
  Reset -> Alarm_Off : [StateCnt>50]
  RestartCounter -> greenState : [RestartCounter < 10]
  data: StateCnt local uint16; iAlarm input boolean; iReset input boolean; oShutoff output boolean; oCurrentAlarm output boolean; RestartCounter local uint8

== stateflow chart BVH2_Appl_Layer/Subsystem/BVH2_Appl_Layer/UbatHandling ==
  state Ubat_Handling [parallel]
    state NormalUbat
      entry:
      odPumpOff          = 0 ;
      odFixedValueSel  = 0 ;
      odPI_Disable       = 0 ;
      oUbat_Alarm_High = 0 ;
      oUbat_Alarm_Low  =  0 ;
    note: iUbat < 5.8V
    state SaturationHigh
      entry:
      odPumpOff = 1 ;
      odFixedValueSel = 0 ;
      odPI_Disable = 0 ;
      oUbat_Alarm_High = 1 ;
      oUbat_Alarm_Low = 0;
    state SaturationLow
      entry:
      odPumpOff = 1 ;
      odFixedValueSel = 0 ;
      odPI_Disable = 0 ;
      oUbat_Alarm_High = 1 ;
      oUbat_Alarm_Low = 1 ;
    note: iUbat > 28V
    note: iUbat < 27V
    note: iUbat > 6.3V
    (junction 44) -> NormalUbat
    (default) -> NormalUbat : [iReset==1]
    (junction 44) -> SaturationLow : [iUbat<UbatThresLimpLow-2]
    SaturationLow -> (junction 44) : [iUbat>UbatThresLimpLow+2]
    NormalUbat -> (junction 44)
    SaturationHigh -> (junction 44) : [ iUbat<UbatThresMax - 8]
    (junction 44) -> SaturationHigh : [ iUbat>UbatThresMax]
  data: iUbat input uint8; odFixedValueSel output boolean; odPumpOff output boolean; odPI_Disable output boolean; oUbat_Alarm_High output boolean; oUbat_Alarm_Low output boolean; UbatThresMax constant uint8 =230; UbatThresLimpHigh constant uint8 =63; UbatThresMin constant uint8 =40; iReset input uint8; UbatThresLimpLow constant uint8 =47

== stateflow chart BVH2_Appl_Layer/Subsystem/BVH2_Appl_Layer/Temperature_Alarm ==
  state greenTemp
    entry:
    oTempRedAlarm = 0 ;
    oTempAlarm = 0 ;
    odPumpOff = 0;
    Counter = 0;
  state reset
    entry:
    Counter = 0;
  state CntOverTemp
    during:
    Counter++;
  note: iTemp < 75°C
  note: iTemp > 110°C
  state redTemp
    entry:
    oTempRedAlarm = 1 ;
    oTempAlarm = 1 ;
    odPumpOff = 0; // test
  note: Wait for 400ms after reset
  CntOverTemp -> greenTemp : [Counter > 80   ]
  greenTemp -> redTemp : [iTemp < Treshold_red  ]
  reset -> CntOverTemp
  (default) -> reset : [iReset==1]
  redTemp -> greenTemp : [iTemp> Treshold_green   ]
  data: iTemp input uint16; oTempRedAlarm output boolean; Treshold_red constant uint16 =72; iReset input boolean; oTempAlarm output boolean; Treshold_green constant uint16 =185; Threshold_RedAlarm constant uint16 =72; odPumpOff output boolean; Counter local uint8

== stateflow chart BVH2_Appl_Layer/Subsystem/BVH2_Appl_Layer/Pic_etat_monitor ==
  state redState
    entry:
    StateCnt=0;
    oShutoff = 1;
    oAlarm = 1;
  state Wrong_ETAT
    entry:
    StateCnt = 0 ;
    during:
    StateCnt++ ;
  state Alarm_Off
    entry:
    oShutoff  = 0 ;
    oAlarm = 0;
  state Reset
    entry:
    StateCnt=0;
    during:
    StateCnt++ ;
  state greenState
    entry:
    oShutoff  = 0 ;
    oAlarm = 0;
    StateCnt = 0;
    during:
    StateCnt++;
  state Wait
    entry:
    StateCnt = 0;
    during:
    StateCnt++;
  (junction 95) -> Wrong_ETAT : [iAlarm==1]
  (default) -> Reset : [iReset==1]
  redState -> Wait : [iAlarm == 0]
  (junction 94) -> redState : [StateCnt  > 0]
  Wrong_ETAT -> (junction 94)
  (junction 94) -> Alarm_Off : [iAlarm == 0]
  Reset -> greenState : [StateCnt>50]
  Alarm_Off -> (junction 95)
  greenState -> (junction 95)
  (junction 95) -> Alarm_Off : [ StateCnt  > 5 ]
  (junction 96) -> greenState : [StateCnt  > 15]
  (junction 96) -> redState : [iAlarm == 1]
  Wait -> (junction 96)
  data: StateCnt local uint16; iAlarm input boolean; iReset input boolean; oShutoff output boolean; oAlarm output boolean

== stateflow chart BVH2_Appl_Layer/Subsystem/BVH2_Appl_Layer/Current_Analysis_low ==
  state redState
    entry:
    oShutoff = 0;
    oCurrentAlarm = 1 ;
  state CntOverCurrent
    entry:
    StateCnt = 0 ;
    during:
    StateCnt++ ;
  state greenState
    entry:
    oShutoff    = 0 ;
    oCurrentAlarm = 0 ;
  state Wait
    entry:
    StateCnt = 0;
    during:
    StateCnt++;
  note: iCurrent > 9A
  note: iCurrent > 9A
  note: iCurrent < 9A
  note: iCurrent < 9A
  note: Use the typical values (offset compensate) for BTN8962.
  note: /* When the current is over 9A,
      | for 250ms,
      | an alarm in generated. */
  greenState -> CntOverCurrent : [iCurrent>iThreshold-2]
  (default) -> greenState : [iReset==1]
  (junction 127) -> greenState : [iCurrent< iThreshold+2]
  (junction 127) -> redState : [StateCnt  > 50]
  CntOverCurrent -> (junction 127)
  redState -> Wait : [iCurrent< iThreshold+2]
  Wait -> (junction 128)
  (junction 128) -> greenState : [StateCnt  > 100]
  (junction 128) -> redState : [iCurrent>iThreshold-2]
  data: iCurrent input uint16; oShutoff output boolean; iReset input uint8; oCurrentAlarm output boolean; StateCnt local uint8; iThreshold input uint16 =182

== stateflow chart BVH2_Appl_Layer/Subsystem/BVH2_Appl_Layer/Dry_Running ==
  state greenState
    entry:
    oDryRunAlarm = 0 ;
  note: Dry running is detected when the current is
      | below 2,0A (low speed) and 3,8A (high speed)
  state DryRunning
    state redState
      entry:
      oDryRunAlarm = 1 ;
    state CntOverCurrent
      entry:
      StateCnt = 0 ;
      oDryRunAlarm = 0 ;
      during:
      StateCnt++ ;
    (junction 152) -> redState : [StateCnt  > 2000]
    CntOverCurrent -> (junction 152)
  note: iSpeed = 400 => 2000rpm
      | iSpeed = 80 => 10000rpm
  greenState -> CntOverCurrent : [(iCurrent ) < iThreshold-5 && iSpeed < 400 && iSpeed > 80 ]
  (default) -> greenState : [iReset==1]
  (junction 152) -> greenState : [iPWM < 20 && iPWM > 4]
  (junction 152) -> greenState : [(iCurrent) > iThreshold+5 || iSpeed > 400 || iSpeed < 80 ]
  data: iPWM input double; iReset input uint8; oDryRunAlarm output boolean; StateCnt local uint16; iCurrent input uint16; iSpeed input uint16; iThreshold input uint16 =8548

== stateflow chart BVH2_Appl_Layer/Subsystem/BVH2_Appl_Layer/Motor_Stalled ==
  state default
    entry:
    oMotorStalled=0 ;
    oStalledAlarm = 0 ;
    RestartCounter = 0
  state Motor_stalled_Statemachine
    state SpeedBad_cnt
      entry:
      oStalledAlarm = 0  ;
      StateCnt = 0;
      during:
      BadCnt++ ;
      StateCnt++ ;
    state Speed_detection
      during:
      StateCnt++ ;
    state CntStart
      entry:
      StateCnt = 0  ;
      BadCnt = 0 ;
      during:
      StateCnt++ ;
      exit:
      StateCnt = 0 ;
    state Motor_Stalled
      entry:
      StateCnt = 0 ;
      oMotorStalled=1;
      oStalledAlarm= 1 ;
      during:
      StateCnt++
    state Motor_Run
      entry:
      StateCnt=0 ;
      BadCnt = 0 ;
      oMotorStalled=0;
      oStalledAlarm = 0 ;
      // Detection allways
    state Motor_Wait
      entry:
      StateCnt = 0 ;
      oMotorStalled=0;
      oStalledAlarm= 1;
      RestartCounter ++;
      during:
      StateCnt++;
    note: 2670 rpm < iSpeed < 170000 rpm
    (junction 179) -> Speed_detection : [iSpeed >= TresholdLow_Speed && iSpeed <= ThresholdHigh_Speed]
    Speed_detection -> (junction 178)
    (junction 178) -> Motor_Run : [StateCnt > 1000]
    CntStart -> Speed_detection : [ (StateCnt) > 0   ]
    (junction 179) -> Motor_Stalled : [BadCnt>100]
    (junction 178) -> SpeedBad_cnt : [iSpeed < TresholdLow_Speed || iSpeed > ThresholdHigh_Speed ]
    SpeedBad_cnt -> (junction 179)
    Motor_Stalled -> Motor_Wait : [ StateCnt > 200 ]
    (junction 180) -> Motor_Stalled : [iSpeed < TresholdLow_Speed || iSpeed > ThresholdHigh_Speed ]
    (junction 180) -> Motor_Run : [StateCnt > 200]
    Motor_Wait -> (junction 180) : [StateCnt > 10]
    Motor_Run -> Speed_detection
  state Stop
    entry:
    oStalledAlarm = 1;
    oMotorStalled = 1;
  Motor_stalled_Statemachine -> default : [ iMotor_off == true || Reset == true ]
  default -> CntStart : [iMotor_off == false ]
  (default) -> default : [Reset == true]
  (junction 180) -> Stop : [RestartCounter == 10]
  data: iMotor_off input boolean; StateCnt local uint16; TresholdLow_Speed constant uint16 =5; oMotorStalled output boolean; BadCnt local uint16; Reset input boolean; iSpeed input uint16; oStalledAlarm output boolean; false constant boolean; true constant boolean =1; ThresholdHigh_Speed constant uint16 =300; RestartCounter local uint8; iCurrentAlarm input boolean

== stateflow chart BVH2_Appl_Layer/Subsystem/BVH2_Appl_Layer/PWM_Detection ==
  state PWMinput_handling [parallel]
    state PumpOff2
      entry:
      odPumpOff          = 1 ;
      odFixedValueSel  = 0 ;
      odFixedLowValueSel = 0 ;
      odPI_Disable       = 1 ;
      oPWM_SC_Alarm = 0 ;
      oPWM_Alarm  =  0 ;
    state Normal3
      entry:
      odPumpOff      = 0 ;
      odFixedLowValueSel = 0 ;
      odFixedValueSel = 0 ;
      odPI_Disable   = 0 ;
      oPWM_SC_Alarm = 0 ;
      oPWM_Alarm  =  0 ;
    state LimpModeLow
      entry:
      odPumpOff = 0 ;
      odFixedValueSel = 1 ;
      odFixedLowValueSel = 0 ;
      odPI_Disable = 0 ;
      oPWM_SC_Alarm = 1 ;
      oPWM_Alarm = 0 ;
    state Notice that between 90 -94 % [group]
      Input PWM duty cylcle the maximum
      output PWM duty cycle is limited (saturated)
      outside this statmachine
    state SaturationHigh
      entry:
      odPumpOff = 0 ;
      odFixedValueSel = 1 ;
      odFixedLowValueSel = 0 ;
      odPI_Disable = 0 ;
      oPWM_SC_Alarm = 1 ;
      oPWM_Alarm = 0 ;
    state SaturationLow
      entry:
      odPumpOff      = 0 ;
      odFixedValueSel = 0 ;
      odFixedLowValueSel = 1 ;
      odPI_Disable   = 0 ;
      oPWM_SC_Alarm = 0 ;
      oPWM_Alarm  =  0 ;
    state Alarm
      entry:
      odPumpOff = 0 ;
      odFixedValueSel = 1 ;
      odFixedLowValueSel = 0 ;
      odPI_Disable = 0 ;
      oPWM_SC_Alarm = 1 ;
      oPWM_Alarm = 0 ;
    state CMD_MJP_0_100
      entry:
      odPumpOff = 0 ;
      odFixedValueSel = 1 ;
      odFixedLowValueSel = 0 ;
      odPI_Disable = 0 ;
      oPWM_SC_Alarm = 0 ;
      oPWM_Alarm = 1 ;
    state LimpModeLow1
      entry:
      odPumpOff = 1 ;
      odFixedValueSel = 0 ;
      odFixedLowValueSel = 0 ;
      odPI_Disable = 0 ;
      oPWM_SC_Alarm = 1 ;
      oPWM_Alarm = 0 ;
    Normal3 -> (junction 222)
    (default) -> PumpOff2 : [iReset==1]
    (junction 222) -> Normal3 : [(idPWM>=23)]
    (junction 222) -> PumpOff2 : [(idPWM<=19)]
    PumpOff2 -> (junction 222)
    LimpModeLow -> (junction 222)
    (junction 222) -> LimpModeLow : [ (idPWM <= 5 ) ]
    (junction 222) -> SaturationHigh : [ ( idPWM > 191) ]
    SaturationHigh -> (junction 222)
    (junction 222) -> SaturationLow : [(idPWM>19)]
    SaturationLow -> (junction 222)
    (junction 222) -> Alarm : [(( iPWM_Freq < Low_Freq ) || ( iPWM_Freq > High_Freq ))]
    Alarm -> (junction 222)
    CMD_MJP_0_100 -> (junction 222)
    (junction 222) -> CMD_MJP_0_100 : [ (idPWM < 1) || (idPWM > 199) ]
    (junction 222) -> LimpModeLow1 : [ (idPWM < 9) ]
    LimpModeLow1 -> (junction 222)
  data: iPWM_Freq input uint16; idPWM input uint8; DTCs local uint8 size=8; odFixedValueSel output boolean; odPumpOff output boolean; index local uint8; DTC local uint8; NDTC local uint8 =8; NoDTC local boolean =1; TempDTC local uint8; WAITTIME constant uint8 =25; count local uint8; SavedDTC local uint8; odPI_Disable output boolean; ST7_Ready local boolean; oPWM_SC_Alarm output boolean; oPWM_Alarm output boolean; iReset input uint8; odFixedLowValueSel output boolean; Low_Freq constant uint16 =36000; High_Freq constant uint16 =44000
  data DTCs settings: description=$TL$ name=$O; class=STATIC_LOCAL; $TL$
  data DTC settings: description=$TL$ name=$O; class=GLOBAL; $TL$
  data NDTC settings: description=$TL$ name=$O; class=CONST; $TL$
  data ST7_Ready settings: description=$TL$ name=$O; class=GLOBAL; $TL$
